simulink model "Simulink_6"  (R2016b)
settings: Solver=VariableStepAuto  StartTime=0.0  StopTime=70  RelTol=1e-3
values from neighbouring files (symbols this model uses):
  C_lon = [1 0 0 0 ... (first row only)    [ejercicio07_longitudinal_C.m]
  D_lon = zeros(2)    [ejercicio07_longitudinal_C.m]
  delta_e_dot_lim = [-90 90]    [ejercicio07_lateral_C.m]    (also in ejercicio07_longitudinal_C.m)
  delta_e_lim = [-25 25]    [ejercicio07_lateral_C.m]    (also in ejercicio07_longitudinal_C.m)
  delta_th_dot_lim = [-0.24 0.24]*100    [ejercicio07_lateral_C.m]    (also in ejercicio07_longitudinal_C.m)
  delta_th_lim = [-0.2 0.8]*100    [ejercicio07_lateral_C.m]    (also in ejercicio07_longitudinal_C.m)
  dt = 0.001    [ejercicio07_lateral_C.m]    (also in ejercicio07_longitudinal_C.m)
  F_lon = A_lon*Tm + I    [ejercicio07_longitudinal_C.m]
  G_lon = B_lon*Tm    [ejercicio07_longitudinal_C.m]
  Kc = Kc_a(:,1:4)    [ejercicio07_lateral_C.m]    (also in ejercicio07_longitudinal_C.m)
  Ki = -Kc_a(:,5:6)    [ejercicio07_lateral_C.m]    (also in ejercicio07_longitudinal_C.m)
  Ko_d = dlqe(F_lat,G_lat,C_lat,V1,V2)    [ejercicio07_lateral_C.m]    (also in ejercicio07_longitudinal_C.m = dlqe(F_lon,G_lon,C_lon,V1,V2))
  PreC = [Cyr*(I-Fyr)^(-1)*G_lat+D_lat]^(-1)    [ejercicio07_lateral_C.m]    (also in ejercicio07_longitudinal_C.m = [Cyr*(I-Fyr)^(-1)*G_lon+D_lon]^(-1))
  tau_e = 1/20    (= 0.05)    [ejercicio07_longitudinal_C.m]
  tau_th = 0.5    [ejercicio07_longitudinal_C.m]
  Tm = 0.003    [ejercicio07_lateral_C.m]    (also in ejercicio07_longitudinal_C.m)
undefined symbols (not defined in the file or in its folder): DiscIntNeverNeededParam, Ko
undefined symbols (not defined in the file): sys_lon
(part 2 of 3)

== system Simulink_6/Ejercicio 6/EJERCICIO 6 DISCRETO/Comparativa ejercicio 6/Comparativa Integral/CONTROL LONGITUDINAL CONTINUO ACCION INTEGRAL ==
  ACTUADORES : Subsystem
  Add : Sum  Inputs=+
  Add1 : Sum  Inputs=+
  Add2 : Sum  Inputs=+
  DINAMICA LONGITUDINAL : Subsystem  mask(Dinámica longitudinal F-16){A=sys_lon.a, B=sys_lon.b, C=sys_lon.c, D=sys_lon.d, X0=[0 0 0 0]}
      mask prompts: A "Matriz de estados (A)"; B "Matriz de entrada (B)"; C "Matriz de salida (C)"; D "Matriz de transmisión directa (D)"; X0 "Condiciones iniciales (nominales)"
      mask help: Modelo lineal de la dinámica longitudinal del F-16
  FILTRO SP : Subsystem
  Gain1 : Gain  Gain=PreC  Multiplication=Matrix(K*u)
  KT/taup2 : Gain  Gain=Kc  Multiplication=Matrix(K*u)
  Mux : Mux  Inputs=2
  OBSERVADOR : Subsystem  mask(Dinámica longitudinal F-16){A=sys_lon.a, B=sys_lon.b, C=sys_lon.c, D=sys_lon.d, X0=[0 0 0 0], Ko=Ko}
      mask prompts: A "Matriz de estados (A)"; B "Matriz de entrada (B)"; C "Matriz de salida (C)"; D "Matriz de transmisión directa (D)"; X0 "Condiciones iniciales (nominales)"; Ko "Ganancia del observador"
      mask help: Modelo lineal de la dinámica longitudinal del F-16
  Perturbación1 : Step  Time=[45 46]  After=[1 -1]*3  SampleTime=0
  SENSORES : Subsystem
  Sum1 : Sum  Inputs=|+-
  Sum2 : Sum  Inputs=|++
  Sum3 : Sum  Inputs=|+-
  Transfer Fcn : TransferFcn  Denominator=[1 1]
  thetaSP1 : Step  Time=[35,40]  Before=[0,0]  After=[5,5]  SampleTime=0
  vT_SP1 : Step  Time=[1,20]  Before=[0,0]  After=[30,15]  SampleTime=0
  CONTINUA : Outport
  wires:
  Add1/1 -> FILTRO SP/1(vt-sp)
  Gain1/1 -> Sum1/1
  Add2/1 -> FILTRO SP/2(theta_sp)
  thetaSP1/1 -> Add2/1
  DINAMICA LONGITUDINAL/1(y) -> Mux/1, SENSORES/1(y)  "y"
  [SP] -> Mux/2
  SENSORES/1(ym) -> OBSERVADOR/2(y), Sum3/2
  Mux/1 -> CONTINUA/1
  Perturbación1/1 -> Add/1
  OBSERVADOR/1(xest) -> KT/taup2/1
  Sum1/1 -> ACTUADORES/1(e)
  vT_SP1/1 -> Add1/1
  ACTUADORES/1(u) -> OBSERVADOR/1(u), Sum2/2
  Sum2/1 -> DINAMICA LONGITUDINAL/1(u)
  KT/taup2/1 -> Sum1/2
  Add/1 -> Transfer Fcn/1
  Transfer Fcn/1 -> Sum2/1
  Sum3/1 -> Gain1/1
  FILTRO SP/1(sp) -> Sum3/1, [SP]

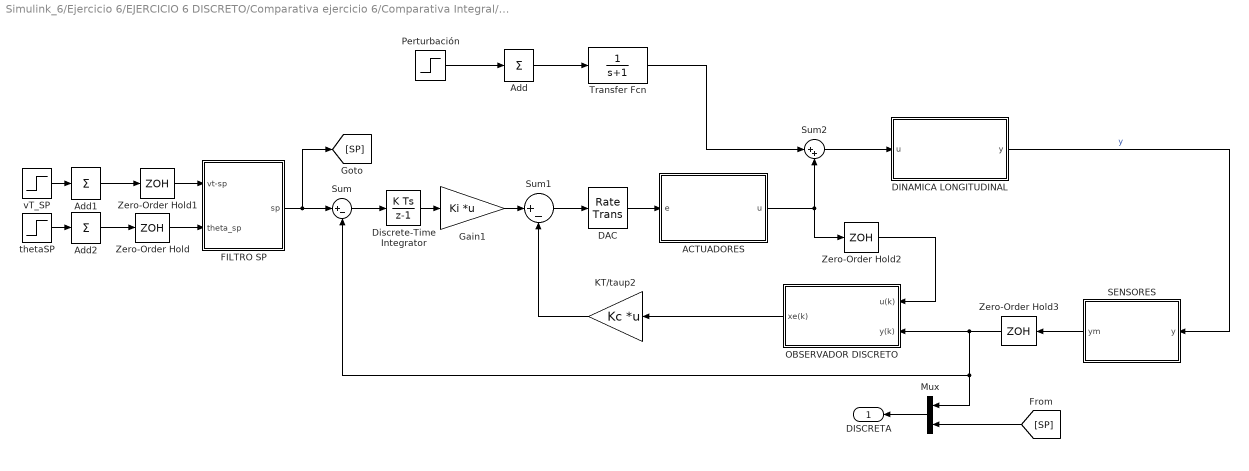
== system Simulink_6/Ejercicio 6/EJERCICIO 6 DISCRETO/Comparativa ejercicio 6/Comparativa Integral/CONTROL LONGITUDINAL DISCRETO ACCION INTEGRAL ==
  ACTUADORES : Subsystem
  Add : Sum  Inputs=+
  Add1 : Sum  Inputs=+
  Add2 : Sum  Inputs=+
  DAC : RateTransition  OutPortSampleTime=Tm
  DINAMICA LONGITUDINAL : Subsystem  mask(Dinámica longitudinal F-16){A=sys_lon.a, B=sys_lon.b, C=sys_lon.c, D=sys_lon.d, X0=[0 0 0 0]}
      mask prompts: A "Matriz de estados (A)"; B "Matriz de entrada (B)"; C "Matriz de salida (C)"; D "Matriz de transmisión directa (D)"; X0 "Condiciones iniciales (nominales)"
      mask help: Modelo lineal de la dinámica longitudinal del F-16
  Discrete-Time Integrator : DiscreteIntegrator  InitialConditionSetting=State (most efficient)  SampleTime=-1  ICPrevOutput=DiscIntNeverNeededParam  ICPrevScaledInput=DiscIntNeverNeededParam
  FILTRO SP : Subsystem
  Gain1 : Gain  Gain=Ki  Multiplication=Matrix(K*u)
  KT/taup2 : Gain  Gain=Kc  Multiplication=Matrix(K*u)
  Mux : Mux  Inputs=2
  OBSERVADOR DISCRETO : Subsystem  mask(Dinámica longitudinal F-16){F=F_lon, G=G_lon, C=C_lon, D=D_lon, Ko=Ko_d}
      mask prompts: F "Matriz de estados (A)"; G "Matriz de entrada (B)"; C "Matriz de salida (C)"; D "Matriz de transmisión directa (D)"; Ko "Ganancia del observador"
      mask help: Modelo lineal de la dinámica longitudinal del F-16
  Perturbación : Step  Time=[45 46]  After=[1 -1]*3  SampleTime=0
  SENSORES : Subsystem
  Sum : Sum  Inputs=|+-
  Sum1 : Sum  Inputs=|+-
  Sum2 : Sum  Inputs=|++
  Transfer Fcn : TransferFcn  Denominator=[1 1]
  Zero-Order Hold{,1..3} (4 alike) : ZeroOrderHold  SampleTime=-1
  thetaSP : Step  Time=[35,40]  Before=[0,0]  After=[5,5]  SampleTime=0
  vT_SP : Step  Time=[1,20]  Before=[0,0]  After=[30,15]  SampleTime=0
  DISCRETA : Outport
  wires:
  Zero-Order Hold/1 -> FILTRO SP/2(theta_sp)
  ACTUADORES/1(u) -> Sum2/2, Zero-Order Hold2/1
  Add/1 -> Transfer Fcn/1
  FILTRO SP/1(sp) -> Sum/1, [SP]
  DAC/1 -> ACTUADORES/1(e)
  Mux/1 -> DISCRETA/1
  OBSERVADOR DISCRETO/1(xe(k)) -> KT/taup2/1
  DINAMICA LONGITUDINAL/1(y) -> SENSORES/1(y)  "y"
  Transfer Fcn/1 -> Sum2/1
  KT/taup2/1 -> Sum1/2
  Zero-Order Hold2/1 -> OBSERVADOR DISCRETO/1(u(k))
  SENSORES/1(ym) -> Zero-Order Hold3/1
  Zero-Order Hold3/1 -> OBSERVADOR DISCRETO/2(y(k)), Sum/2, Mux/1
  [SP] -> Mux/2
  Add1/1 -> Zero-Order Hold1/1
  Add2/1 -> Zero-Order Hold/1
  Sum2/1 -> DINAMICA LONGITUDINAL/1(u)
  Sum1/1 -> DAC/1
  Zero-Order Hold1/1 -> FILTRO SP/1(vt-sp)
  vT_SP/1 -> Add1/1
  Perturbación/1 -> Add/1
  thetaSP/1 -> Add2/1
  Gain1/1 -> Sum1/1
  Sum/1 -> Discrete-Time Integrator/1
  Discrete-Time Integrator/1 -> Gain1/1

== system Simulink_6/Ejercicio 6/EJERCICIO 6 DISCRETO/Comparativa ejercicio 6/Comparativa modal/CONTROL LONGITUDINAL CONTINUA ==
  ACTUADORES : Subsystem
  Add : Sum  Inputs=+
  Add1 : Sum  Inputs=+
  Add2 : Sum  Inputs=+
  DINAMICA LONGITUDINAL : Subsystem  mask(Dinámica longitudinal F-16){A=sys_lon.a, B=sys_lon.b, C=sys_lon.c, D=sys_lon.d, X0=[0 0 0 0]}
      mask prompts: A "Matriz de estados (A)"; B "Matriz de entrada (B)"; C "Matriz de salida (C)"; D "Matriz de transmisión directa (D)"; X0 "Condiciones iniciales (nominales)"
      mask help: Modelo lineal de la dinámica longitudinal del F-16
  FILTRO SP : Subsystem
  Gain1 : Gain  Gain=PreC  Multiplication=Matrix(K*u)
  KT/taup2 : Gain  Gain=Kc  Multiplication=Matrix(K*u)
  Mux : Mux  Inputs=2
  OBSERVADOR : Subsystem  mask(Dinámica longitudinal F-16){A=sys_lon.a, B=sys_lon.b, C=sys_lon.c, D=sys_lon.d, X0=[0 0 0 0], Ko=Ko}
      mask prompts: A "Matriz de estados (A)"; B "Matriz de entrada (B)"; C "Matriz de salida (C)"; D "Matriz de transmisión directa (D)"; X0 "Condiciones iniciales (nominales)"; Ko "Ganancia del observador"
      mask help: Modelo lineal de la dinámica longitudinal del F-16
  Perturbación1 : Step  Time=[45 46]  After=[1 -1]*3  SampleTime=0
  SENSORES : Subsystem
  Sum1 : Sum  Inputs=|+-
  Sum2 : Sum  Inputs=|++
  Transfer Fcn : TransferFcn  Denominator=[1 1]
  thetaSP1 : Step  Time=[35,40]  Before=[0,0]  After=[5,5]  SampleTime=0
  vT_SP1 : Step  Time=[1,20]  Before=[0,0]  After=[30,15]  SampleTime=0
  CONTINUA : Outport
  wires:
  OBSERVADOR/1(xest) -> KT/taup2/1
  [SP] -> Mux/2
  vT_SP1/1 -> Add1/1
  Add2/1 -> FILTRO SP/2(theta_sp)
  thetaSP1/1 -> Add2/1
  Sum1/1 -> ACTUADORES/1(e)
  DINAMICA LONGITUDINAL/1(y) -> Mux/1, SENSORES/1(y)  "y"
  SENSORES/1(ym) -> OBSERVADOR/2(y)
  Gain1/1 -> Sum1/1
  KT/taup2/1 -> Sum1/2
  Add1/1 -> FILTRO SP/1(vt-sp)
  Add/1 -> Transfer Fcn/1
  Perturbación1/1 -> Add/1
  Sum2/1 -> DINAMICA LONGITUDINAL/1(u)
  Transfer Fcn/1 -> Sum2/1
  ACTUADORES/1(u) -> OBSERVADOR/1(u), Sum2/2
  FILTRO SP/1(sp) -> Gain1/1, [SP]
  Mux/1 -> CONTINUA/1

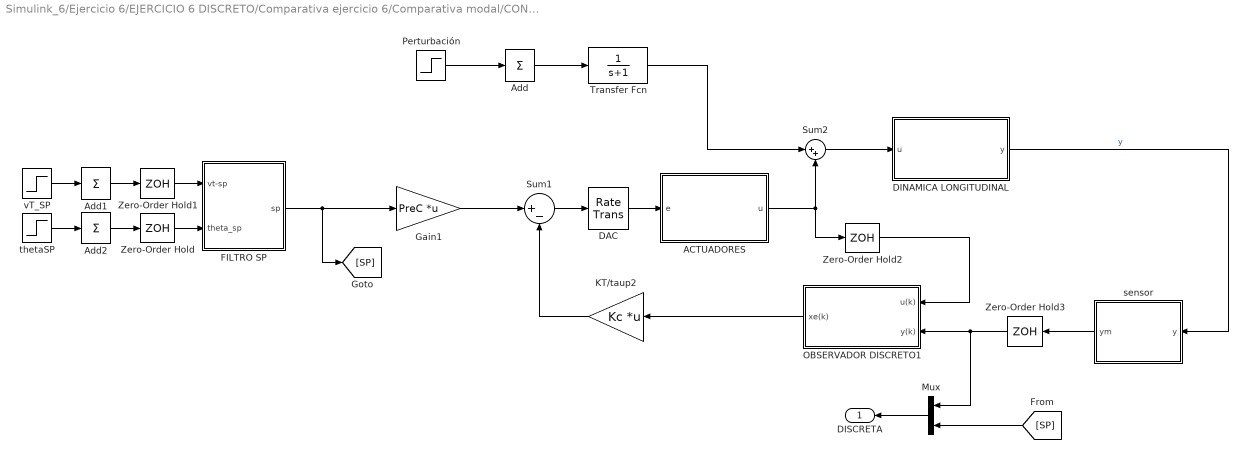
== system Simulink_6/Ejercicio 6/EJERCICIO 6 DISCRETO/Comparativa ejercicio 6/Comparativa modal/CONTROL LONGITUDINAL DISCRETO ==
  ACTUADORES : Subsystem
  Add : Sum  Inputs=+
  Add1 : Sum  Inputs=+
  Add2 : Sum  Inputs=+
  DAC : RateTransition  OutPortSampleTime=Tm
  DINAMICA LONGITUDINAL : Subsystem  mask(Dinámica longitudinal F-16){A=sys_lon.a, B=sys_lon.b, C=sys_lon.c, D=sys_lon.d, X0=[0 0 0 0]}
      mask prompts: A "Matriz de estados (A)"; B "Matriz de entrada (B)"; C "Matriz de salida (C)"; D "Matriz de transmisión directa (D)"; X0 "Condiciones iniciales (nominales)"
      mask help: Modelo lineal de la dinámica longitudinal del F-16
  FILTRO SP : Subsystem
  Gain1 : Gain  Gain=PreC  Multiplication=Matrix(K*u)
  KT/taup2 : Gain  Gain=Kc  Multiplication=Matrix(K*u)
  Mux : Mux  Inputs=2
  OBSERVADOR DISCRETO1 : Subsystem  mask(Dinámica longitudinal F-16){F=F_lon, G=G_lon, C=C_lon, D=D_lon, Ko=Ko_d}
      mask prompts: F "Matriz de estados (A)"; G "Matriz de entrada (B)"; C "Matriz de salida (C)"; D "Matriz de transmisión directa (D)"; Ko "Ganancia del observador"
      mask help: Modelo lineal de la dinámica longitudinal del F-16
  Perturbación : Step  Time=[45 46]  After=[1 -1]*3  SampleTime=0
  Sum1 : Sum  Inputs=|+-
  Sum2 : Sum  Inputs=|++
  Transfer Fcn : TransferFcn  Denominator=[1 1]
  Zero-Order Hold{,1..3} (4 alike) : ZeroOrderHold  SampleTime=-1
  sensor : Subsystem
  thetaSP : Step  Time=[35,40]  Before=[0,0]  After=[5,5]  SampleTime=0
  vT_SP : Step  Time=[1,20]  Before=[0,0]  After=[30,15]  SampleTime=0
  DISCRETA : Outport
  wires:
  KT/taup2/1 -> Sum1/2
  FILTRO SP/1(sp) -> Gain1/1, [SP]
  Gain1/1 -> Sum1/1
  OBSERVADOR DISCRETO1/1(xe(k)) -> KT/taup2/1
  Mux/1 -> DISCRETA/1
  [SP] -> Mux/2
  ACTUADORES/1(u) -> Zero-Order Hold2/1, Sum2/2
  Sum2/1 -> DINAMICA LONGITUDINAL/1(u)
  Transfer Fcn/1 -> Sum2/1
  Add/1 -> Transfer Fcn/1
  Perturbación/1 -> Add/1
  thetaSP/1 -> Add2/1
  vT_SP/1 -> Add1/1
  Add2/1 -> Zero-Order Hold/1
  Zero-Order Hold1/1 -> FILTRO SP/1(vt-sp)
  Add1/1 -> Zero-Order Hold1/1
  Zero-Order Hold/1 -> FILTRO SP/2(theta_sp)
  DAC/1 -> ACTUADORES/1(e)
  Sum1/1 -> DAC/1
  Zero-Order Hold2/1 -> OBSERVADOR DISCRETO1/1(u(k))
  DINAMICA LONGITUDINAL/1(y) -> sensor/1(y)  "y"
  sensor/1(ym) -> Zero-Order Hold3/1
  Zero-Order Hold3/1 -> OBSERVADOR DISCRETO1/2(y(k)), Mux/1

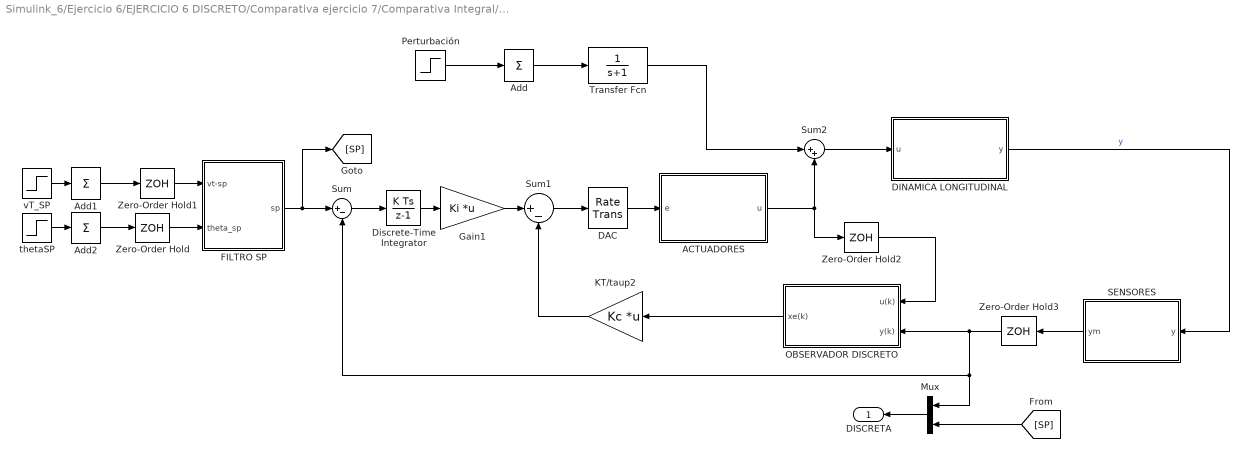
== system Simulink_6/Ejercicio 6/EJERCICIO 6 DISCRETO/Comparativa ejercicio 7/Comparativa Integral/CONTROL LONGITUDINAL DISCRETO ACCION INTEGRAL ==
  ACTUADORES : Subsystem
  Add : Sum  Inputs=+
  Add1 : Sum  Inputs=+
  Add2 : Sum  Inputs=+
  DAC : RateTransition  OutPortSampleTime=Tm
  DINAMICA LONGITUDINAL : Subsystem  mask(Dinámica longitudinal F-16){A=sys_lon.a, B=sys_lon.b, C=sys_lon.c, D=sys_lon.d, X0=[0 0 0 0]}
      mask prompts: A "Matriz de estados (A)"; B "Matriz de entrada (B)"; C "Matriz de salida (C)"; D "Matriz de transmisión directa (D)"; X0 "Condiciones iniciales (nominales)"
      mask help: Modelo lineal de la dinámica longitudinal del F-16
  Discrete-Time Integrator : DiscreteIntegrator  InitialConditionSetting=State (most efficient)  SampleTime=-1  ICPrevOutput=DiscIntNeverNeededParam  ICPrevScaledInput=DiscIntNeverNeededParam
  FILTRO SP : Subsystem
  Gain1 : Gain  Gain=Ki  Multiplication=Matrix(K*u)
  KT/taup2 : Gain  Gain=Kc  Multiplication=Matrix(K*u)
  Mux : Mux  Inputs=2
  OBSERVADOR DISCRETO : Subsystem  mask(Dinámica longitudinal F-16){F=F_lon, G=G_lon, C=C_lon, D=D_lon, Ko=Ko_d}
      mask prompts: F "Matriz de estados (A)"; G "Matriz de entrada (B)"; C "Matriz de salida (C)"; D "Matriz de transmisión directa (D)"; Ko "Ganancia del observador"
      mask help: Modelo lineal de la dinámica longitudinal del F-16
  Perturbación : Step  Time=[45 46]  After=[1 -1]*3  SampleTime=0
  SENSORES : Subsystem
  Sum : Sum  Inputs=|+-
  Sum1 : Sum  Inputs=|+-
  Sum2 : Sum  Inputs=|++
  Transfer Fcn : TransferFcn  Denominator=[1 1]
  Zero-Order Hold{,1..3} (4 alike) : ZeroOrderHold  SampleTime=-1
  thetaSP : Step  Time=[35,40]  Before=[0,0]  After=[5,5]  SampleTime=0
  vT_SP : Step  Time=[1,20]  Before=[0,0]  After=[30,15]  SampleTime=0
  DISCRETA : Outport
  wires:
  Zero-Order Hold/1 -> FILTRO SP/2(theta_sp)
  ACTUADORES/1(u) -> Sum2/2, Zero-Order Hold2/1
  Add/1 -> Transfer Fcn/1
  FILTRO SP/1(sp) -> Sum/1, [SP]
  DAC/1 -> ACTUADORES/1(e)
  Mux/1 -> DISCRETA/1
  OBSERVADOR DISCRETO/1(xe(k)) -> KT/taup2/1
  DINAMICA LONGITUDINAL/1(y) -> SENSORES/1(y)  "y"
  Transfer Fcn/1 -> Sum2/1
  KT/taup2/1 -> Sum1/2
  Zero-Order Hold2/1 -> OBSERVADOR DISCRETO/1(u(k))
  SENSORES/1(ym) -> Zero-Order Hold3/1
  Zero-Order Hold3/1 -> OBSERVADOR DISCRETO/2(y(k)), Sum/2, Mux/1
  [SP] -> Mux/2
  Add1/1 -> Zero-Order Hold1/1
  Add2/1 -> Zero-Order Hold/1
  Sum2/1 -> DINAMICA LONGITUDINAL/1(u)
  Sum1/1 -> DAC/1
  Zero-Order Hold1/1 -> FILTRO SP/1(vt-sp)
  vT_SP/1 -> Add1/1
  Perturbación/1 -> Add/1
  thetaSP/1 -> Add2/1
  Gain1/1 -> Sum1/1
  Sum/1 -> Discrete-Time Integrator/1
  Discrete-Time Integrator/1 -> Gain1/1

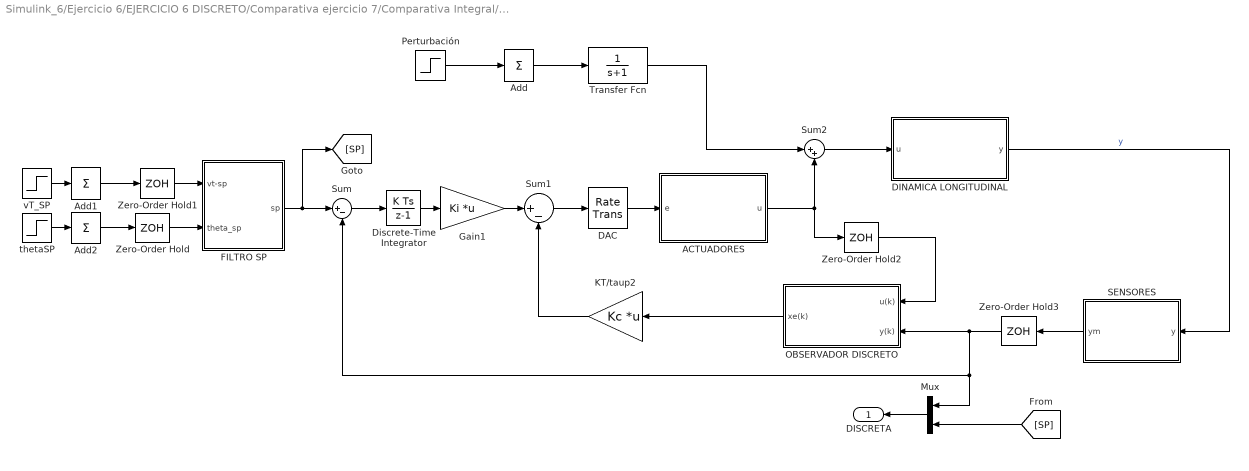
== system Simulink_6/Ejercicio 6/EJERCICIO 6 DISCRETO/Comparativa ejercicio 7/Comparativa Integral/CONTROL LONGITUDINAL DISCRETO ACCION INTEGRAL1 ==
  ACTUADORES : Subsystem
  Add : Sum  Inputs=+
  Add1 : Sum  Inputs=+
  Add2 : Sum  Inputs=+
  DAC : RateTransition  OutPortSampleTime=Tm
  DINAMICA LONGITUDINAL : Subsystem  mask(Dinámica longitudinal F-16){A=sys_lon.a, B=sys_lon.b, C=sys_lon.c, D=sys_lon.d, X0=[0 0 0 0]}
      mask prompts: A "Matriz de estados (A)"; B "Matriz de entrada (B)"; C "Matriz de salida (C)"; D "Matriz de transmisión directa (D)"; X0 "Condiciones iniciales (nominales)"
      mask help: Modelo lineal de la dinámica longitudinal del F-16
  Discrete-Time Integrator : DiscreteIntegrator  InitialConditionSetting=State (most efficient)  SampleTime=-1  ICPrevOutput=DiscIntNeverNeededParam  ICPrevScaledInput=DiscIntNeverNeededParam
  FILTRO SP : Subsystem
  Gain1 : Gain  Gain=Ki  Multiplication=Matrix(K*u)
  KT/taup2 : Gain  Gain=Kc  Multiplication=Matrix(K*u)
  Mux : Mux  Inputs=2
  OBSERVADOR DISCRETO : Subsystem  mask(Dinámica longitudinal F-16){F=F_lon, G=G_lon, C=C_lon, D=D_lon, Ko=Ko_d}
      mask prompts: F "Matriz de estados (A)"; G "Matriz de entrada (B)"; C "Matriz de salida (C)"; D "Matriz de transmisión directa (D)"; Ko "Ganancia del observador"
      mask help: Modelo lineal de la dinámica longitudinal del F-16
  Perturbación : Step  Time=[45 46]  After=[1 -1]*3  SampleTime=0
  SENSORES : Subsystem
  Sum : Sum  Inputs=|+-
  Sum1 : Sum  Inputs=|+-
  Sum2 : Sum  Inputs=|++
  Transfer Fcn : TransferFcn  Denominator=[1 1]
  Zero-Order Hold{,1..3} (4 alike) : ZeroOrderHold  SampleTime=-1
  thetaSP : Step  Time=[35,40]  Before=[0,0]  After=[5,5]  SampleTime=0
  vT_SP : Step  Time=[1,20]  Before=[0,0]  After=[30,15]  SampleTime=0
  DISCRETA : Outport
  wires:
  Zero-Order Hold/1 -> FILTRO SP/2(theta_sp)
  ACTUADORES/1(u) -> Sum2/2, Zero-Order Hold2/1
  Add/1 -> Transfer Fcn/1
  FILTRO SP/1(sp) -> Sum/1, [SP]
  DAC/1 -> ACTUADORES/1(e)
  Mux/1 -> DISCRETA/1
  OBSERVADOR DISCRETO/1(xe(k)) -> KT/taup2/1
  DINAMICA LONGITUDINAL/1(y) -> SENSORES/1(y)  "y"
  Transfer Fcn/1 -> Sum2/1
  KT/taup2/1 -> Sum1/2
  Zero-Order Hold2/1 -> OBSERVADOR DISCRETO/1(u(k))
  SENSORES/1(ym) -> Zero-Order Hold3/1
  Zero-Order Hold3/1 -> OBSERVADOR DISCRETO/2(y(k)), Sum/2, Mux/1
  [SP] -> Mux/2
  Add1/1 -> Zero-Order Hold1/1
  Add2/1 -> Zero-Order Hold/1
  Sum2/1 -> DINAMICA LONGITUDINAL/1(u)
  Sum1/1 -> DAC/1
  Zero-Order Hold1/1 -> FILTRO SP/1(vt-sp)
  vT_SP/1 -> Add1/1
  Perturbación/1 -> Add/1
  thetaSP/1 -> Add2/1
  Gain1/1 -> Sum1/1
  Sum/1 -> Discrete-Time Integrator/1
  Discrete-Time Integrator/1 -> Gain1/1

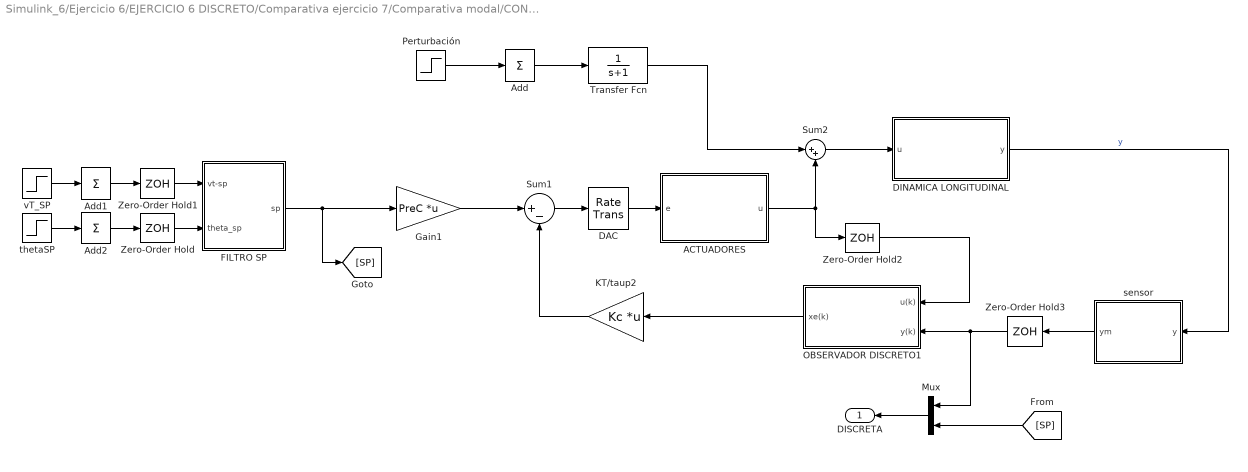
== system Simulink_6/Ejercicio 6/EJERCICIO 6 DISCRETO/Comparativa ejercicio 7/Comparativa modal/CONTROL LONGITUDINAL DISCRETO EJERCICIO 6 ==
  ACTUADORES : Subsystem
  Add : Sum  Inputs=+
  Add1 : Sum  Inputs=+
  Add2 : Sum  Inputs=+
  DAC : RateTransition  OutPortSampleTime=Tm
  DINAMICA LONGITUDINAL : Subsystem  mask(Dinámica longitudinal F-16){A=sys_lon.a, B=sys_lon.b, C=sys_lon.c, D=sys_lon.d, X0=[0 0 0 0]}
      mask prompts: A "Matriz de estados (A)"; B "Matriz de entrada (B)"; C "Matriz de salida (C)"; D "Matriz de transmisión directa (D)"; X0 "Condiciones iniciales (nominales)"
      mask help: Modelo lineal de la dinámica longitudinal del F-16
  FILTRO SP : Subsystem
  Gain1 : Gain  Gain=PreC  Multiplication=Matrix(K*u)
  KT/taup2 : Gain  Gain=Kc  Multiplication=Matrix(K*u)
  Mux : Mux  Inputs=2
  OBSERVADOR DISCRETO1 : Subsystem  mask(Dinámica longitudinal F-16){F=F_lon, G=G_lon, C=C_lon, D=D_lon, Ko=Ko_d}
      mask prompts: F "Matriz de estados (A)"; G "Matriz de entrada (B)"; C "Matriz de salida (C)"; D "Matriz de transmisión directa (D)"; Ko "Ganancia del observador"
      mask help: Modelo lineal de la dinámica longitudinal del F-16
  Perturbación : Step  Time=[45 46]  After=[1 -1]*3  SampleTime=0
  Sum1 : Sum  Inputs=|+-
  Sum2 : Sum  Inputs=|++
  Transfer Fcn : TransferFcn  Denominator=[1 1]
  Zero-Order Hold{,1..3} (4 alike) : ZeroOrderHold  SampleTime=-1
  sensor : Subsystem
  thetaSP : Step  Time=[35,40]  Before=[0,0]  After=[5,5]  SampleTime=0
  vT_SP : Step  Time=[1,20]  Before=[0,0]  After=[30,15]  SampleTime=0
  DISCRETA : Outport
  wires:
  KT/taup2/1 -> Sum1/2
  FILTRO SP/1(sp) -> Gain1/1, [SP]
  Gain1/1 -> Sum1/1
  OBSERVADOR DISCRETO1/1(xe(k)) -> KT/taup2/1
  Mux/1 -> DISCRETA/1
  [SP] -> Mux/2
  ACTUADORES/1(u) -> Zero-Order Hold2/1, Sum2/2
  Sum2/1 -> DINAMICA LONGITUDINAL/1(u)
  Transfer Fcn/1 -> Sum2/1
  Add/1 -> Transfer Fcn/1
  Perturbación/1 -> Add/1
  thetaSP/1 -> Add2/1
  vT_SP/1 -> Add1/1
  Add2/1 -> Zero-Order Hold/1
  Zero-Order Hold1/1 -> FILTRO SP/1(vt-sp)
  Add1/1 -> Zero-Order Hold1/1
  Zero-Order Hold/1 -> FILTRO SP/2(theta_sp)
  DAC/1 -> ACTUADORES/1(e)
  Sum1/1 -> DAC/1
  Zero-Order Hold2/1 -> OBSERVADOR DISCRETO1/1(u(k))
  DINAMICA LONGITUDINAL/1(y) -> sensor/1(y)  "y"
  sensor/1(ym) -> Zero-Order Hold3/1
  Zero-Order Hold3/1 -> OBSERVADOR DISCRETO1/2(y(k)), Mux/1

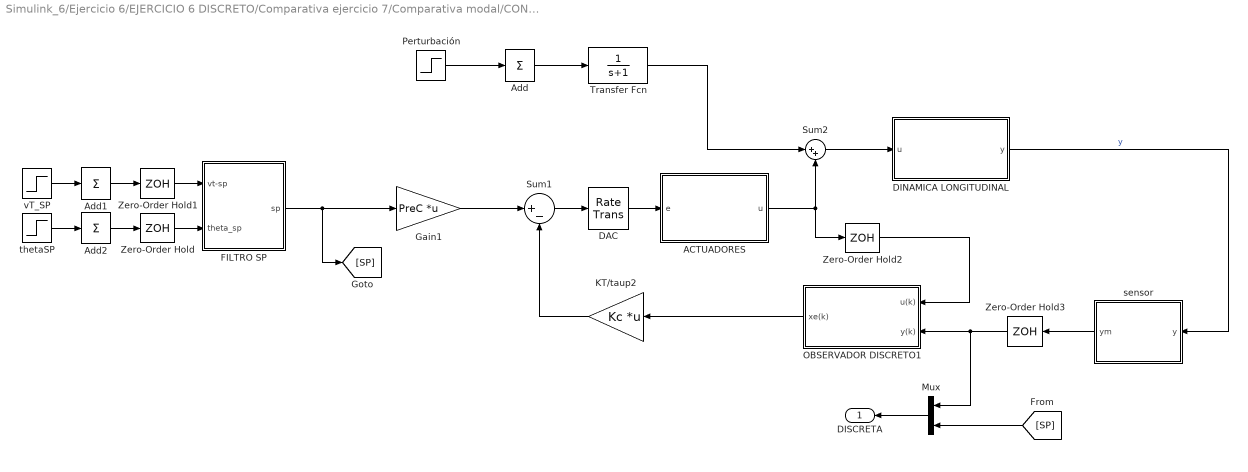
== system Simulink_6/Ejercicio 6/EJERCICIO 6 DISCRETO/Comparativa ejercicio 7/Comparativa modal/CONTROL LONGITUDINAL DISCRETO EJERCICIO 7 ==
  ACTUADORES : Subsystem
  Add : Sum  Inputs=+
  Add1 : Sum  Inputs=+
  Add2 : Sum  Inputs=+
  DAC : RateTransition  OutPortSampleTime=Tm
  DINAMICA LONGITUDINAL : Subsystem  mask(Dinámica longitudinal F-16){A=sys_lon.a, B=sys_lon.b, C=sys_lon.c, D=sys_lon.d, X0=[0 0 0 0]}
      mask prompts: A "Matriz de estados (A)"; B "Matriz de entrada (B)"; C "Matriz de salida (C)"; D "Matriz de transmisión directa (D)"; X0 "Condiciones iniciales (nominales)"
      mask help: Modelo lineal de la dinámica longitudinal del F-16
  FILTRO SP : Subsystem
  Gain1 : Gain  Gain=PreC  Multiplication=Matrix(K*u)
  KT/taup2 : Gain  Gain=Kc  Multiplication=Matrix(K*u)
  Mux : Mux  Inputs=2
  OBSERVADOR DISCRETO1 : Subsystem  mask(Dinámica longitudinal F-16){F=F_lon, G=G_lon, C=C_lon, D=D_lon, Ko=Ko_d}
      mask prompts: F "Matriz de estados (A)"; G "Matriz de entrada (B)"; C "Matriz de salida (C)"; D "Matriz de transmisión directa (D)"; Ko "Ganancia del observador"
      mask help: Modelo lineal de la dinámica longitudinal del F-16
  Perturbación : Step  Time=[45 46]  After=[1 -1]*3  SampleTime=0
  Sum1 : Sum  Inputs=|+-
  Sum2 : Sum  Inputs=|++
  Transfer Fcn : TransferFcn  Denominator=[1 1]
  Zero-Order Hold{,1..3} (4 alike) : ZeroOrderHold  SampleTime=-1
  sensor : Subsystem
  thetaSP : Step  Time=[35,40]  Before=[0,0]  After=[5,5]  SampleTime=0
  vT_SP : Step  Time=[1,20]  Before=[0,0]  After=[30,15]  SampleTime=0
  DISCRETA : Outport
  wires:
  KT/taup2/1 -> Sum1/2
  FILTRO SP/1(sp) -> Gain1/1, [SP]
  Gain1/1 -> Sum1/1
  OBSERVADOR DISCRETO1/1(xe(k)) -> KT/taup2/1
  Mux/1 -> DISCRETA/1
  [SP] -> Mux/2
  ACTUADORES/1(u) -> Zero-Order Hold2/1, Sum2/2
  Sum2/1 -> DINAMICA LONGITUDINAL/1(u)
  Transfer Fcn/1 -> Sum2/1
  Add/1 -> Transfer Fcn/1
  Perturbación/1 -> Add/1
  thetaSP/1 -> Add2/1
  vT_SP/1 -> Add1/1
  Add2/1 -> Zero-Order Hold/1
  Zero-Order Hold1/1 -> FILTRO SP/1(vt-sp)
  Add1/1 -> Zero-Order Hold1/1
  Zero-Order Hold/1 -> FILTRO SP/2(theta_sp)
  DAC/1 -> ACTUADORES/1(e)
  Sum1/1 -> DAC/1
  Zero-Order Hold2/1 -> OBSERVADOR DISCRETO1/1(u(k))
  DINAMICA LONGITUDINAL/1(y) -> sensor/1(y)  "y"
  sensor/1(ym) -> Zero-Order Hold3/1
  Zero-Order Hold3/1 -> OBSERVADOR DISCRETO1/2(y(k)), Mux/1

== system Simulink_6/Ejercicio 6/EJERCICIO 6 DISCRETO/Comparativa ejercicio 6/Comparativa Integral/CONTROL LONGITUDINAL CONTINUO ACCION INTEGRAL/ACTUADORES ==
  e : Inport
  Actuadores : Scope
  Demux : Demux  Outputs=2
  ELEVADOR : Subsystem
  Gain4 : Gain  Gain=[1 180/pi]
  Mux1 : Mux  Inputs=2
  THROTTLE : Subsystem
  u : Outport
  wires:
  Demux/1 -> THROTTLE/1(u_th)
  Demux/2 -> ELEVADOR/1(u_e)
  ELEVADOR/1(delta_e) -> Mux1/2
  e/1 -> Demux/1
  Mux1/1 -> u/1, Gain4/1
  Gain4/1 -> Actuadores/1
  THROTTLE/1(delta_th) -> Mux1/1

== system Simulink_6/Ejercicio 6/EJERCICIO 6 DISCRETO/Comparativa ejercicio 6/Comparativa Integral/CONTROL LONGITUDINAL CONTINUO ACCION INTEGRAL/DINAMICA LONGITUDINAL ==
  u : Inport
  Integrator5 : Integrator
  Km1 : Gain  Gain=D  Multiplication=Matrix(K*u)
  Km10 : Gain  Gain=A  Multiplication=Matrix(K*u)
  Km2 : Gain  Gain=C  Multiplication=Matrix(K*u)
  Km8 : Gain  Gain=B  Multiplication=Matrix(K*u)
  Sum1 : Sum  Inputs=++|
  Sum12 : Sum  Inputs=|++
  y : Outport
  wires:
  Km8/1 -> Sum12/1
  Sum12/1 -> Integrator5/1
  Integrator5/1 -> Km2/1, Km10/1  "x"
  Km10/1 -> Sum12/2
  Km2/1 -> Sum1/2
  Km1/1 -> Sum1/1
  Sum1/1 -> y/1
  u/1 -> Km8/1, Km1/1

== system Simulink_6/Ejercicio 6/EJERCICIO 6 DISCRETO/Comparativa ejercicio 6/Comparativa Integral/CONTROL LONGITUDINAL CONTINUO ACCION INTEGRAL/FILTRO SP ==
  vt-sp : Inport
  theta_sp : Inport  Port=2
  Mux4 : Mux  Inputs=2
  Rate Limiter : RateLimiter  RisingSlewLimit=3  FallingSlewLimit=-3  SampleTimeMode=inherited
  Transfer Fcn : TransferFcn  Denominator=[1 1]
  sp : Outport
  wires:
  Rate Limiter/1 -> Transfer Fcn/1
  Transfer Fcn/1 -> Mux4/1
  vt-sp/1 -> Rate Limiter/1
  Mux4/1 -> sp/1
  theta_sp/1 -> Mux4/2

== system Simulink_6/Ejercicio 6/EJERCICIO 6 DISCRETO/Comparativa ejercicio 6/Comparativa Integral/CONTROL LONGITUDINAL CONTINUO ACCION INTEGRAL/OBSERVADOR ==
  u : Inport
  y : Inport  Port=2
  Integrator5 : Integrator
  Km1 : Gain  Gain=D  Multiplication=Matrix(K*u)
  Km10 : Gain  Gain=A  Multiplication=Matrix(K*u)
  Km2 : Gain  Gain=C  Multiplication=Matrix(K*u)
  Km3 : Gain  Gain=Ko  Multiplication=Matrix(K*u)
  Km8 : Gain  Gain=B  Multiplication=Matrix(K*u)
  Sum1 : Sum  Inputs=++|
  Sum12 : Sum  Inputs=+++
  Sum2 : Sum  Inputs=+-|
  xest : Outport
  wires:
  Km8/1 -> Sum12/1
  Sum12/1 -> Integrator5/1
  Integrator5/1 -> Km2/1, Km10/1, xest/1  "xe"
  Km10/1 -> Sum12/3
  Km2/1 -> Sum1/2
  Km1/1 -> Sum1/1
  Sum1/1 -> Sum2/2  "ye"
  u/1 -> Km8/1, Km1/1
  y/1 -> Sum2/1
  Sum2/1 -> Km3/1
  Km3/1 -> Sum12/2

== system Simulink_6/Ejercicio 6/EJERCICIO 6 DISCRETO/Comparativa ejercicio 6/Comparativa Integral/CONTROL LONGITUDINAL CONTINUO ACCION INTEGRAL/SENSORES ==
  y : Inport
  Add2 : Sum
  Add3 : Sum
  Demux : Demux  Outputs=2
  Mux2 : Mux  Inputs=2
  Ruido de medida1 : RandomNumber  Variance=1e-6  Seed=123456  SampleTime=dt
  Ruido de medida2 : RandomNumber  Variance=1e-6  Seed=123456  SampleTime=dt
  ym : Outport
  wires:
  y/1 -> Demux/1
  Ruido de medida1/1 -> Add2/1
  Add2/1 -> Mux2/1
  Demux/1 -> Add2/2
  Mux2/1 -> ym/1
  Demux/2 -> Add3/1
  Add3/1 -> Mux2/2
  Ruido de medida2/1 -> Add3/2

== system Simulink_6/Ejercicio 6/EJERCICIO 6 DISCRETO/Comparativa ejercicio 6/Comparativa Integral/CONTROL LONGITUDINAL DISCRETO ACCION INTEGRAL/ACTUADORES ==
  e : Inport
  Actuadores : Scope
  Demux : Demux  Outputs=2
  ELEVADOR : Subsystem
  Gain4 : Gain  Gain=[1 180/pi]
  Mux1 : Mux  Inputs=2
  THROTTLE : Subsystem
  u : Outport
  wires:
  Demux/1 -> THROTTLE/1(u_th)
  Demux/2 -> ELEVADOR/1(u_e)
  ELEVADOR/1(delta_e) -> Mux1/2
  e/1 -> Demux/1
  Mux1/1 -> u/1, Gain4/1
  Gain4/1 -> Actuadores/1
  THROTTLE/1(delta_th) -> Mux1/1

== system Simulink_6/Ejercicio 6/EJERCICIO 6 DISCRETO/Comparativa ejercicio 6/Comparativa Integral/CONTROL LONGITUDINAL DISCRETO ACCION INTEGRAL/DINAMICA LONGITUDINAL ==
  u : Inport
  Integrator5 : Integrator
  Km1 : Gain  Gain=D  Multiplication=Matrix(K*u)
  Km10 : Gain  Gain=A  Multiplication=Matrix(K*u)
  Km2 : Gain  Gain=C  Multiplication=Matrix(K*u)
  Km8 : Gain  Gain=B  Multiplication=Matrix(K*u)
  Sum1 : Sum  Inputs=++|
  Sum12 : Sum  Inputs=|++
  y : Outport
  wires:
  Km8/1 -> Sum12/1
  Sum12/1 -> Integrator5/1
  Integrator5/1 -> Km2/1, Km10/1  "x"
  Km10/1 -> Sum12/2
  Km2/1 -> Sum1/2
  Km1/1 -> Sum1/1
  Sum1/1 -> y/1
  u/1 -> Km8/1, Km1/1

== system Simulink_6/Ejercicio 6/EJERCICIO 6 DISCRETO/Comparativa ejercicio 6/Comparativa Integral/CONTROL LONGITUDINAL DISCRETO ACCION INTEGRAL/FILTRO SP ==
  vt-sp : Inport
  theta_sp : Inport  Port=2
  Discrete Transfer Fcn : DiscreteTransferFcn  Numerator=[Tm]  Denominator=[1 -1+Tm]
  Mux4 : Mux  Inputs=2
  Rate Limiter : RateLimiter  RisingSlewLimit=3  FallingSlewLimit=-3  SampleTimeMode=inherited
  sp : Outport
  wires:
  vt-sp/1 -> Rate Limiter/1
  Mux4/1 -> sp/1
  theta_sp/1 -> Mux4/2
  Rate Limiter/1 -> Discrete Transfer Fcn/1
  Discrete Transfer Fcn/1 -> Mux4/1

== system Simulink_6/Ejercicio 6/EJERCICIO 6 DISCRETO/Comparativa ejercicio 6/Comparativa Integral/CONTROL LONGITUDINAL DISCRETO ACCION INTEGRAL/OBSERVADOR DISCRETO ==
  u(k) : Inport
  y(k) : Inport  Port=2
  Km1 : Gain  Gain=D  Multiplication=Matrix(K*u)
  Km10 : Gain  Gain=F  Multiplication=Matrix(K*u)
  Km2 : Gain  Gain=C  Multiplication=Matrix(K*u)
  Km3 : Gain  Gain=Ko  Multiplication=Matrix(K*u)
  Km8 : Gain  Gain=G  Multiplication=Matrix(K*u)
  Sum1 : Sum  Inputs=++|
  Sum12 : Sum  Inputs=+++
  Sum2 : Sum  Inputs=+-|
  Unit Delay : UnitDelay  SampleTime=Tm  HasFrameUpgradeWarning=on
  xe(k) : Outport
  wires:
  Km8/1 -> Sum12/1
  Sum12/1 -> Unit Delay/1  "xe(k+1)"
  Unit Delay/1 -> Km2/1, Km10/1, xe(k)/1  "xe(k)"
  Km10/1 -> Sum12/3
  Km2/1 -> Sum1/2
  Km1/1 -> Sum1/1
  Sum1/1 -> Sum2/2  "ye(k)"
  u(k)/1 -> Km8/1, Km1/1
  y(k)/1 -> Sum2/1
  Sum2/1 -> Km3/1
  Km3/1 -> Sum12/2

== system Simulink_6/Ejercicio 6/EJERCICIO 6 DISCRETO/Comparativa ejercicio 6/Comparativa Integral/CONTROL LONGITUDINAL DISCRETO ACCION INTEGRAL/SENSORES ==
  y : Inport
  Add2 : Sum
  Add3 : Sum
  Demux : Demux  Outputs=2
  Mux2 : Mux  Inputs=2
  Ruido de medida1 : RandomNumber  Variance=1e-6  Seed=123456  SampleTime=dt
  Ruido de medida2 : RandomNumber  Variance=1e-6  Seed=123456  SampleTime=dt
  ym : Outport
  wires:
  y/1 -> Demux/1
  Ruido de medida1/1 -> Add2/1
  Add2/1 -> Mux2/1
  Demux/1 -> Add2/2
  Mux2/1 -> ym/1
  Demux/2 -> Add3/1
  Add3/1 -> Mux2/2
  Ruido de medida2/1 -> Add3/2

== system Simulink_6/Ejercicio 6/EJERCICIO 6 DISCRETO/Comparativa ejercicio 6/Comparativa modal/CONTROL LONGITUDINAL CONTINUA/ACTUADORES ==
  e : Inport
  Actuadores : Scope
  Demux : Demux  Outputs=2
  ELEVADOR : Subsystem
  Gain4 : Gain  Gain=[1 180/pi]
  Mux1 : Mux  Inputs=2
  THROTTLE : Subsystem
  u : Outport
  wires:
  Demux/1 -> THROTTLE/1(u_th)
  Demux/2 -> ELEVADOR/1(u_e)
  ELEVADOR/1(delta_e) -> Mux1/2
  e/1 -> Demux/1
  Mux1/1 -> u/1, Gain4/1
  Gain4/1 -> Actuadores/1
  THROTTLE/1(delta_th) -> Mux1/1

== system Simulink_6/Ejercicio 6/EJERCICIO 6 DISCRETO/Comparativa ejercicio 6/Comparativa modal/CONTROL LONGITUDINAL CONTINUA/DINAMICA LONGITUDINAL ==
  u : Inport
  Integrator5 : Integrator
  Km1 : Gain  Gain=D  Multiplication=Matrix(K*u)
  Km10 : Gain  Gain=A  Multiplication=Matrix(K*u)
  Km2 : Gain  Gain=C  Multiplication=Matrix(K*u)
  Km8 : Gain  Gain=B  Multiplication=Matrix(K*u)
  Sum1 : Sum  Inputs=++|
  Sum12 : Sum  Inputs=|++
  y : Outport
  wires:
  Km8/1 -> Sum12/1
  Sum12/1 -> Integrator5/1
  Integrator5/1 -> Km2/1, Km10/1  "x"
  Km10/1 -> Sum12/2
  Km2/1 -> Sum1/2
  Km1/1 -> Sum1/1
  Sum1/1 -> y/1
  u/1 -> Km8/1, Km1/1

== system Simulink_6/Ejercicio 6/EJERCICIO 6 DISCRETO/Comparativa ejercicio 6/Comparativa modal/CONTROL LONGITUDINAL CONTINUA/FILTRO SP ==
  vt-sp : Inport
  theta_sp : Inport  Port=2
  Mux4 : Mux  Inputs=2
  Rate Limiter : RateLimiter  RisingSlewLimit=3  FallingSlewLimit=-3  SampleTimeMode=inherited
  Transfer Fcn : TransferFcn  Denominator=[1 1]
  sp : Outport
  wires:
  Rate Limiter/1 -> Transfer Fcn/1
  Transfer Fcn/1 -> Mux4/1
  vt-sp/1 -> Rate Limiter/1
  Mux4/1 -> sp/1
  theta_sp/1 -> Mux4/2

== system Simulink_6/Ejercicio 6/EJERCICIO 6 DISCRETO/Comparativa ejercicio 6/Comparativa modal/CONTROL LONGITUDINAL CONTINUA/OBSERVADOR ==
  u : Inport
  y : Inport  Port=2
  Integrator5 : Integrator
  Km1 : Gain  Gain=D  Multiplication=Matrix(K*u)
  Km10 : Gain  Gain=A  Multiplication=Matrix(K*u)
  Km2 : Gain  Gain=C  Multiplication=Matrix(K*u)
  Km3 : Gain  Gain=Ko  Multiplication=Matrix(K*u)
  Km8 : Gain  Gain=B  Multiplication=Matrix(K*u)
  Sum1 : Sum  Inputs=++|
  Sum12 : Sum  Inputs=+++
  Sum2 : Sum  Inputs=+-|
  xest : Outport
  wires:
  Km8/1 -> Sum12/1
  Sum12/1 -> Integrator5/1
  Integrator5/1 -> Km2/1, Km10/1, xest/1  "xe"
  Km10/1 -> Sum12/3
  Km2/1 -> Sum1/2
  Km1/1 -> Sum1/1
  Sum1/1 -> Sum2/2  "ye"
  u/1 -> Km8/1, Km1/1
  y/1 -> Sum2/1
  Sum2/1 -> Km3/1
  Km3/1 -> Sum12/2

== system Simulink_6/Ejercicio 6/EJERCICIO 6 DISCRETO/Comparativa ejercicio 6/Comparativa modal/CONTROL LONGITUDINAL CONTINUA/SENSORES ==
  y : Inport
  Add2 : Sum
  Add3 : Sum
  Demux : Demux  Outputs=2
  Mux2 : Mux  Inputs=2
  Ruido de medida1 : RandomNumber  Variance=1e-6  Seed=123456  SampleTime=dt
  Ruido de medida2 : RandomNumber  Variance=1e-6  Seed=123456  SampleTime=dt
  ym : Outport
  wires:
  y/1 -> Demux/1
  Ruido de medida1/1 -> Add2/1
  Add2/1 -> Mux2/1
  Demux/1 -> Add2/2
  Mux2/1 -> ym/1
  Demux/2 -> Add3/1
  Add3/1 -> Mux2/2
  Ruido de medida2/1 -> Add3/2

== system Simulink_6/Ejercicio 6/EJERCICIO 6 DISCRETO/Comparativa ejercicio 6/Comparativa modal/CONTROL LONGITUDINAL DISCRETO/ACTUADORES ==
  e : Inport
  Actuadores : Scope
  Demux : Demux  Outputs=2
  ELEVADOR : Subsystem
  Gain4 : Gain  Gain=[1 180/pi]
  Mux1 : Mux  Inputs=2
  THROTTLE : Subsystem
  u : Outport
  wires:
  Demux/1 -> THROTTLE/1(u_th)
  Demux/2 -> ELEVADOR/1(u_e)
  ELEVADOR/1(delta_e) -> Mux1/2
  e/1 -> Demux/1
  Mux1/1 -> u/1, Gain4/1
  Gain4/1 -> Actuadores/1
  THROTTLE/1(delta_th) -> Mux1/1

== system Simulink_6/Ejercicio 6/EJERCICIO 6 DISCRETO/Comparativa ejercicio 6/Comparativa modal/CONTROL LONGITUDINAL DISCRETO/DINAMICA LONGITUDINAL ==
  u : Inport
  Integrator5 : Integrator
  Km1 : Gain  Gain=D  Multiplication=Matrix(K*u)
  Km10 : Gain  Gain=A  Multiplication=Matrix(K*u)
  Km2 : Gain  Gain=C  Multiplication=Matrix(K*u)
  Km8 : Gain  Gain=B  Multiplication=Matrix(K*u)
  Sum1 : Sum  Inputs=++|
  Sum12 : Sum  Inputs=|++
  y : Outport
  wires:
  Km8/1 -> Sum12/1
  Sum12/1 -> Integrator5/1
  Integrator5/1 -> Km2/1, Km10/1  "x"
  Km10/1 -> Sum12/2
  Km2/1 -> Sum1/2
  Km1/1 -> Sum1/1
  Sum1/1 -> y/1
  u/1 -> Km8/1, Km1/1

== system Simulink_6/Ejercicio 6/EJERCICIO 6 DISCRETO/Comparativa ejercicio 6/Comparativa modal/CONTROL LONGITUDINAL DISCRETO/FILTRO SP ==
  vt-sp : Inport
  theta_sp : Inport  Port=2
  Discrete Transfer Fcn : DiscreteTransferFcn  Numerator=[Tm]  Denominator=[1 -1+Tm]
  Mux4 : Mux  Inputs=2
  Rate Limiter : RateLimiter  RisingSlewLimit=3  FallingSlewLimit=-3  SampleTimeMode=inherited
  sp : Outport
  wires:
  Rate Limiter/1 -> Discrete Transfer Fcn/1
  vt-sp/1 -> Rate Limiter/1
  Mux4/1 -> sp/1
  theta_sp/1 -> Mux4/2
  Discrete Transfer Fcn/1 -> Mux4/1

== system Simulink_6/Ejercicio 6/EJERCICIO 6 DISCRETO/Comparativa ejercicio 6/Comparativa modal/CONTROL LONGITUDINAL DISCRETO/OBSERVADOR DISCRETO1 ==
  u(k) : Inport
  y(k) : Inport  Port=2
  Km1 : Gain  Gain=D  Multiplication=Matrix(K*u)
  Km10 : Gain  Gain=F  Multiplication=Matrix(K*u)
  Km2 : Gain  Gain=C  Multiplication=Matrix(K*u)
  Km3 : Gain  Gain=Ko  Multiplication=Matrix(K*u)
  Km8 : Gain  Gain=G  Multiplication=Matrix(K*u)
  Sum1 : Sum  Inputs=++|
  Sum12 : Sum  Inputs=+++
  Sum2 : Sum  Inputs=+-|
  Unit Delay : UnitDelay  SampleTime=Tm  HasFrameUpgradeWarning=on
  xe(k) : Outport
  wires:
  Km8/1 -> Sum12/1
  Sum12/1 -> Unit Delay/1  "xe(k+1)"
  Unit Delay/1 -> Km2/1, Km10/1, xe(k)/1  "xe(k)"
  Km10/1 -> Sum12/3
  Km2/1 -> Sum1/2
  Km1/1 -> Sum1/1
  Sum1/1 -> Sum2/2  "ye(k)"
  u(k)/1 -> Km8/1, Km1/1
  y(k)/1 -> Sum2/1
  Sum2/1 -> Km3/1
  Km3/1 -> Sum12/2

== system Simulink_6/Ejercicio 6/EJERCICIO 6 DISCRETO/Comparativa ejercicio 6/Comparativa modal/CONTROL LONGITUDINAL DISCRETO/sensor ==
  y : Inport
  Add2 : Sum
  Add3 : Sum
  Demux : Demux  Outputs=2
  Mux2 : Mux  Inputs=2
  Ruido de medida1 : RandomNumber  Variance=1e-6  Seed=123456  SampleTime=dt
  Ruido de medida2 : RandomNumber  Variance=1e-6  Seed=123456  SampleTime=dt
  ym : Outport
  wires:
  y/1 -> Demux/1
  Ruido de medida1/1 -> Add2/1
  Add2/1 -> Mux2/1
  Demux/1 -> Add2/2
  Mux2/1 -> ym/1
  Demux/2 -> Add3/1
  Add3/1 -> Mux2/2
  Ruido de medida2/1 -> Add3/2

== system Simulink_6/Ejercicio 6/EJERCICIO 6 DISCRETO/Comparativa ejercicio 7/Comparativa Integral/CONTROL LONGITUDINAL DISCRETO ACCION INTEGRAL/ACTUADORES ==
  e : Inport
  Actuadores : Scope
  Demux : Demux  Outputs=2
  ELEVADOR : Subsystem
  Gain4 : Gain  Gain=[1 180/pi]
  Mux1 : Mux  Inputs=2
  THROTTLE : Subsystem
  u : Outport
  wires:
  Demux/1 -> THROTTLE/1(u_th)
  Demux/2 -> ELEVADOR/1(u_e)
  ELEVADOR/1(delta_e) -> Mux1/2
  e/1 -> Demux/1
  Mux1/1 -> u/1, Gain4/1
  Gain4/1 -> Actuadores/1
  THROTTLE/1(delta_th) -> Mux1/1

== system Simulink_6/Ejercicio 6/EJERCICIO 6 DISCRETO/Comparativa ejercicio 7/Comparativa Integral/CONTROL LONGITUDINAL DISCRETO ACCION INTEGRAL/DINAMICA LONGITUDINAL ==
  u : Inport
  Integrator5 : Integrator
  Km1 : Gain  Gain=D  Multiplication=Matrix(K*u)
  Km10 : Gain  Gain=A  Multiplication=Matrix(K*u)
  Km2 : Gain  Gain=C  Multiplication=Matrix(K*u)
  Km8 : Gain  Gain=B  Multiplication=Matrix(K*u)
  Sum1 : Sum  Inputs=++|
  Sum12 : Sum  Inputs=|++
  y : Outport
  wires:
  Km8/1 -> Sum12/1
  Sum12/1 -> Integrator5/1
  Integrator5/1 -> Km2/1, Km10/1  "x"
  Km10/1 -> Sum12/2
  Km2/1 -> Sum1/2
  Km1/1 -> Sum1/1
  Sum1/1 -> y/1
  u/1 -> Km8/1, Km1/1

== system Simulink_6/Ejercicio 6/EJERCICIO 6 DISCRETO/Comparativa ejercicio 7/Comparativa Integral/CONTROL LONGITUDINAL DISCRETO ACCION INTEGRAL/FILTRO SP ==
  vt-sp : Inport
  theta_sp : Inport  Port=2
  Discrete Transfer Fcn : DiscreteTransferFcn  Numerator=[Tm]  Denominator=[1 -1+Tm]
  Mux4 : Mux  Inputs=2
  Rate Limiter : RateLimiter  RisingSlewLimit=3  FallingSlewLimit=-3  SampleTimeMode=inherited
  sp : Outport
  wires:
  vt-sp/1 -> Rate Limiter/1
  Mux4/1 -> sp/1
  theta_sp/1 -> Mux4/2
  Rate Limiter/1 -> Discrete Transfer Fcn/1
  Discrete Transfer Fcn/1 -> Mux4/1

== system Simulink_6/Ejercicio 6/EJERCICIO 6 DISCRETO/Comparativa ejercicio 7/Comparativa Integral/CONTROL LONGITUDINAL DISCRETO ACCION INTEGRAL/OBSERVADOR DISCRETO ==
  u(k) : Inport
  y(k) : Inport  Port=2
  Km1 : Gain  Gain=D  Multiplication=Matrix(K*u)
  Km10 : Gain  Gain=F  Multiplication=Matrix(K*u)
  Km2 : Gain  Gain=C  Multiplication=Matrix(K*u)
  Km3 : Gain  Gain=Ko  Multiplication=Matrix(K*u)
  Km8 : Gain  Gain=G  Multiplication=Matrix(K*u)
  Sum1 : Sum  Inputs=++|
  Sum12 : Sum  Inputs=+++
  Sum2 : Sum  Inputs=+-|
  Unit Delay : UnitDelay  SampleTime=Tm  HasFrameUpgradeWarning=on
  xe(k) : Outport
  wires:
  Km8/1 -> Sum12/1
  Sum12/1 -> Unit Delay/1  "xe(k+1)"
  Unit Delay/1 -> Km2/1, Km10/1, xe(k)/1  "xe(k)"
  Km10/1 -> Sum12/3
  Km2/1 -> Sum1/2
  Km1/1 -> Sum1/1
  Sum1/1 -> Sum2/2  "ye(k)"
  u(k)/1 -> Km8/1, Km1/1
  y(k)/1 -> Sum2/1
  Sum2/1 -> Km3/1
  Km3/1 -> Sum12/2

== system Simulink_6/Ejercicio 6/EJERCICIO 6 DISCRETO/Comparativa ejercicio 7/Comparativa Integral/CONTROL LONGITUDINAL DISCRETO ACCION INTEGRAL/SENSORES ==
  y : Inport
  Add2 : Sum
  Add3 : Sum
  Demux : Demux  Outputs=2
  Mux2 : Mux  Inputs=2
  Ruido de medida1 : RandomNumber  Variance=1e-6  Seed=123456  SampleTime=dt
  Ruido de medida2 : RandomNumber  Variance=1e-6  Seed=123456  SampleTime=dt
  ym : Outport
  wires:
  y/1 -> Demux/1
  Ruido de medida1/1 -> Add2/1
  Add2/1 -> Mux2/1
  Demux/1 -> Add2/2
  Mux2/1 -> ym/1
  Demux/2 -> Add3/1
  Add3/1 -> Mux2/2
  Ruido de medida2/1 -> Add3/2

== system Simulink_6/Ejercicio 6/EJERCICIO 6 DISCRETO/Comparativa ejercicio 7/Comparativa Integral/CONTROL LONGITUDINAL DISCRETO ACCION INTEGRAL1/ACTUADORES ==
  e : Inport
  Actuadores : Scope
  Demux : Demux  Outputs=2
  ELEVADOR : Subsystem
  Gain4 : Gain  Gain=[1 180/pi]
  Mux1 : Mux  Inputs=2
  THROTTLE : Subsystem
  u : Outport
  wires:
  Demux/1 -> THROTTLE/1(u_th)
  Demux/2 -> ELEVADOR/1(u_e)
  ELEVADOR/1(delta_e) -> Mux1/2
  e/1 -> Demux/1
  Mux1/1 -> u/1, Gain4/1
  Gain4/1 -> Actuadores/1
  THROTTLE/1(delta_th) -> Mux1/1

== system Simulink_6/Ejercicio 6/EJERCICIO 6 DISCRETO/Comparativa ejercicio 7/Comparativa Integral/CONTROL LONGITUDINAL DISCRETO ACCION INTEGRAL1/DINAMICA LONGITUDINAL ==
  u : Inport
  Integrator5 : Integrator
  Km1 : Gain  Gain=D  Multiplication=Matrix(K*u)
  Km10 : Gain  Gain=A  Multiplication=Matrix(K*u)
  Km2 : Gain  Gain=C  Multiplication=Matrix(K*u)
  Km8 : Gain  Gain=B  Multiplication=Matrix(K*u)
  Sum1 : Sum  Inputs=++|
  Sum12 : Sum  Inputs=|++
  y : Outport
  wires:
  Km8/1 -> Sum12/1
  Sum12/1 -> Integrator5/1
  Integrator5/1 -> Km2/1, Km10/1  "x"
  Km10/1 -> Sum12/2
  Km2/1 -> Sum1/2
  Km1/1 -> Sum1/1
  Sum1/1 -> y/1
  u/1 -> Km8/1, Km1/1

== system Simulink_6/Ejercicio 6/EJERCICIO 6 DISCRETO/Comparativa ejercicio 7/Comparativa Integral/CONTROL LONGITUDINAL DISCRETO ACCION INTEGRAL1/FILTRO SP ==
  vt-sp : Inport
  theta_sp : Inport  Port=2
  Discrete Transfer Fcn : DiscreteTransferFcn  Numerator=[Tm]  Denominator=[1 -1+Tm]
  Mux4 : Mux  Inputs=2
  Rate Limiter : RateLimiter  RisingSlewLimit=3  FallingSlewLimit=-3  SampleTimeMode=inherited
  sp : Outport
  wires:
  vt-sp/1 -> Rate Limiter/1
  Mux4/1 -> sp/1
  theta_sp/1 -> Mux4/2
  Rate Limiter/1 -> Discrete Transfer Fcn/1
  Discrete Transfer Fcn/1 -> Mux4/1

== system Simulink_6/Ejercicio 6/EJERCICIO 6 DISCRETO/Comparativa ejercicio 7/Comparativa Integral/CONTROL LONGITUDINAL DISCRETO ACCION INTEGRAL1/OBSERVADOR DISCRETO ==
  u(k) : Inport
  y(k) : Inport  Port=2
  Km1 : Gain  Gain=D  Multiplication=Matrix(K*u)
  Km10 : Gain  Gain=F  Multiplication=Matrix(K*u)
  Km2 : Gain  Gain=C  Multiplication=Matrix(K*u)
  Km3 : Gain  Gain=Ko  Multiplication=Matrix(K*u)
  Km8 : Gain  Gain=G  Multiplication=Matrix(K*u)
  Sum1 : Sum  Inputs=++|
  Sum12 : Sum  Inputs=+++
  Sum2 : Sum  Inputs=+-|
  Unit Delay : UnitDelay  SampleTime=Tm  HasFrameUpgradeWarning=on
  xe(k) : Outport
  wires:
  Km8/1 -> Sum12/1
  Sum12/1 -> Unit Delay/1  "xe(k+1)"
  Unit Delay/1 -> Km2/1, Km10/1, xe(k)/1  "xe(k)"
  Km10/1 -> Sum12/3
  Km2/1 -> Sum1/2
  Km1/1 -> Sum1/1
  Sum1/1 -> Sum2/2  "ye(k)"
  u(k)/1 -> Km8/1, Km1/1
  y(k)/1 -> Sum2/1
  Sum2/1 -> Km3/1
  Km3/1 -> Sum12/2

== system Simulink_6/Ejercicio 6/EJERCICIO 6 DISCRETO/Comparativa ejercicio 7/Comparativa Integral/CONTROL LONGITUDINAL DISCRETO ACCION INTEGRAL1/SENSORES ==
  y : Inport
  Add2 : Sum
  Add3 : Sum
  Demux : Demux  Outputs=2
  Mux2 : Mux  Inputs=2
  Ruido de medida1 : RandomNumber  Variance=1e-6  Seed=123456  SampleTime=dt
  Ruido de medida2 : RandomNumber  Variance=1e-6  Seed=123456  SampleTime=dt
  ym : Outport
  wires:
  y/1 -> Demux/1
  Ruido de medida1/1 -> Add2/1
  Add2/1 -> Mux2/1
  Demux/1 -> Add2/2
  Mux2/1 -> ym/1
  Demux/2 -> Add3/1
  Add3/1 -> Mux2/2
  Ruido de medida2/1 -> Add3/2

== system Simulink_6/Ejercicio 6/EJERCICIO 6 DISCRETO/Comparativa ejercicio 7/Comparativa modal/CONTROL LONGITUDINAL DISCRETO EJERCICIO 6/ACTUADORES ==
  e : Inport
  Actuadores : Scope
  Demux : Demux  Outputs=2
  ELEVADOR : Subsystem
  Gain4 : Gain  Gain=[1 180/pi]
  Mux1 : Mux  Inputs=2
  THROTTLE : Subsystem
  u : Outport
  wires:
  Demux/1 -> THROTTLE/1(u_th)
  Demux/2 -> ELEVADOR/1(u_e)
  ELEVADOR/1(delta_e) -> Mux1/2
  e/1 -> Demux/1
  Mux1/1 -> u/1, Gain4/1
  Gain4/1 -> Actuadores/1
  THROTTLE/1(delta_th) -> Mux1/1

== system Simulink_6/Ejercicio 6/EJERCICIO 6 DISCRETO/Comparativa ejercicio 7/Comparativa modal/CONTROL LONGITUDINAL DISCRETO EJERCICIO 6/DINAMICA LONGITUDINAL ==
  u : Inport
  Integrator5 : Integrator
  Km1 : Gain  Gain=D  Multiplication=Matrix(K*u)
  Km10 : Gain  Gain=A  Multiplication=Matrix(K*u)
  Km2 : Gain  Gain=C  Multiplication=Matrix(K*u)
  Km8 : Gain  Gain=B  Multiplication=Matrix(K*u)
  Sum1 : Sum  Inputs=++|
  Sum12 : Sum  Inputs=|++
  y : Outport
  wires:
  Km8/1 -> Sum12/1
  Sum12/1 -> Integrator5/1
  Integrator5/1 -> Km2/1, Km10/1  "x"
  Km10/1 -> Sum12/2
  Km2/1 -> Sum1/2
  Km1/1 -> Sum1/1
  Sum1/1 -> y/1
  u/1 -> Km8/1, Km1/1

== system Simulink_6/Ejercicio 6/EJERCICIO 6 DISCRETO/Comparativa ejercicio 7/Comparativa modal/CONTROL LONGITUDINAL DISCRETO EJERCICIO 6/FILTRO SP ==
  vt-sp : Inport
  theta_sp : Inport  Port=2
  Discrete Transfer Fcn : DiscreteTransferFcn  Numerator=[Tm]  Denominator=[1 -1+Tm]
  Mux4 : Mux  Inputs=2
  Rate Limiter : RateLimiter  RisingSlewLimit=3  FallingSlewLimit=-3  SampleTimeMode=inherited
  sp : Outport
  wires:
  Rate Limiter/1 -> Discrete Transfer Fcn/1
  vt-sp/1 -> Rate Limiter/1
  Mux4/1 -> sp/1
  theta_sp/1 -> Mux4/2
  Discrete Transfer Fcn/1 -> Mux4/1

== system Simulink_6/Ejercicio 6/EJERCICIO 6 DISCRETO/Comparativa ejercicio 7/Comparativa modal/CONTROL LONGITUDINAL DISCRETO EJERCICIO 6/OBSERVADOR DISCRETO1 ==
  u(k) : Inport
  y(k) : Inport  Port=2
  Km1 : Gain  Gain=D  Multiplication=Matrix(K*u)
  Km10 : Gain  Gain=F  Multiplication=Matrix(K*u)
  Km2 : Gain  Gain=C  Multiplication=Matrix(K*u)
  Km3 : Gain  Gain=Ko  Multiplication=Matrix(K*u)
  Km8 : Gain  Gain=G  Multiplication=Matrix(K*u)
  Sum1 : Sum  Inputs=++|
  Sum12 : Sum  Inputs=+++
  Sum2 : Sum  Inputs=+-|
  Unit Delay : UnitDelay  SampleTime=Tm  HasFrameUpgradeWarning=on
  xe(k) : Outport
  wires:
  Km8/1 -> Sum12/1
  Sum12/1 -> Unit Delay/1  "xe(k+1)"
  Unit Delay/1 -> Km2/1, Km10/1, xe(k)/1  "xe(k)"
  Km10/1 -> Sum12/3
  Km2/1 -> Sum1/2
  Km1/1 -> Sum1/1
  Sum1/1 -> Sum2/2  "ye(k)"
  u(k)/1 -> Km8/1, Km1/1
  y(k)/1 -> Sum2/1
  Sum2/1 -> Km3/1
  Km3/1 -> Sum12/2

== system Simulink_6/Ejercicio 6/EJERCICIO 6 DISCRETO/Comparativa ejercicio 7/Comparativa modal/CONTROL LONGITUDINAL DISCRETO EJERCICIO 6/sensor ==
  y : Inport
  Add2 : Sum
  Add3 : Sum
  Demux : Demux  Outputs=2
  Mux2 : Mux  Inputs=2
  Ruido de medida1 : RandomNumber  Variance=1e-6  Seed=123456  SampleTime=dt
  Ruido de medida2 : RandomNumber  Variance=1e-6  Seed=123456  SampleTime=dt
  ym : Outport
  wires:
  y/1 -> Demux/1
  Ruido de medida1/1 -> Add2/1
  Add2/1 -> Mux2/1
  Demux/1 -> Add2/2
  Mux2/1 -> ym/1
  Demux/2 -> Add3/1
  Add3/1 -> Mux2/2
  Ruido de medida2/1 -> Add3/2

== system Simulink_6/Ejercicio 6/EJERCICIO 6 DISCRETO/Comparativa ejercicio 7/Comparativa modal/CONTROL LONGITUDINAL DISCRETO EJERCICIO 7/ACTUADORES ==
  e : Inport
  Actuadores : Scope
  Demux : Demux  Outputs=2
  ELEVADOR : Subsystem
  Gain4 : Gain  Gain=[1 180/pi]
  Mux1 : Mux  Inputs=2
  THROTTLE : Subsystem
  u : Outport
  wires:
  Demux/1 -> THROTTLE/1(u_th)
  Demux/2 -> ELEVADOR/1(u_e)
  ELEVADOR/1(delta_e) -> Mux1/2
  e/1 -> Demux/1
  Mux1/1 -> u/1, Gain4/1
  Gain4/1 -> Actuadores/1
  THROTTLE/1(delta_th) -> Mux1/1

== system Simulink_6/Ejercicio 6/EJERCICIO 6 DISCRETO/Comparativa ejercicio 7/Comparativa modal/CONTROL LONGITUDINAL DISCRETO EJERCICIO 7/DINAMICA LONGITUDINAL ==
  u : Inport
  Integrator5 : Integrator
  Km1 : Gain  Gain=D  Multiplication=Matrix(K*u)
  Km10 : Gain  Gain=A  Multiplication=Matrix(K*u)
  Km2 : Gain  Gain=C  Multiplication=Matrix(K*u)
  Km8 : Gain  Gain=B  Multiplication=Matrix(K*u)
  Sum1 : Sum  Inputs=++|
  Sum12 : Sum  Inputs=|++
  y : Outport
  wires:
  Km8/1 -> Sum12/1
  Sum12/1 -> Integrator5/1
  Integrator5/1 -> Km2/1, Km10/1  "x"
  Km10/1 -> Sum12/2
  Km2/1 -> Sum1/2
  Km1/1 -> Sum1/1
  Sum1/1 -> y/1
  u/1 -> Km8/1, Km1/1

== system Simulink_6/Ejercicio 6/EJERCICIO 6 DISCRETO/Comparativa ejercicio 7/Comparativa modal/CONTROL LONGITUDINAL DISCRETO EJERCICIO 7/FILTRO SP ==
  vt-sp : Inport
  theta_sp : Inport  Port=2
  Discrete Transfer Fcn : DiscreteTransferFcn  Numerator=[Tm]  Denominator=[1 -1+Tm]
  Mux4 : Mux  Inputs=2
  Rate Limiter : RateLimiter  RisingSlewLimit=3  FallingSlewLimit=-3  SampleTimeMode=inherited
  sp : Outport
  wires:
  Rate Limiter/1 -> Discrete Transfer Fcn/1
  vt-sp/1 -> Rate Limiter/1
  Mux4/1 -> sp/1
  theta_sp/1 -> Mux4/2
  Discrete Transfer Fcn/1 -> Mux4/1

== system Simulink_6/Ejercicio 6/EJERCICIO 6 DISCRETO/Comparativa ejercicio 7/Comparativa modal/CONTROL LONGITUDINAL DISCRETO EJERCICIO 7/OBSERVADOR DISCRETO1 ==
  u(k) : Inport
  y(k) : Inport  Port=2
  Km1 : Gain  Gain=D  Multiplication=Matrix(K*u)
  Km10 : Gain  Gain=F  Multiplication=Matrix(K*u)
  Km2 : Gain  Gain=C  Multiplication=Matrix(K*u)
  Km3 : Gain  Gain=Ko  Multiplication=Matrix(K*u)
  Km8 : Gain  Gain=G  Multiplication=Matrix(K*u)
  Sum1 : Sum  Inputs=++|
  Sum12 : Sum  Inputs=+++
  Sum2 : Sum  Inputs=+-|
  Unit Delay : UnitDelay  SampleTime=Tm  HasFrameUpgradeWarning=on
  xe(k) : Outport
  wires:
  Km8/1 -> Sum12/1
  Sum12/1 -> Unit Delay/1  "xe(k+1)"
  Unit Delay/1 -> Km2/1, Km10/1, xe(k)/1  "xe(k)"
  Km10/1 -> Sum12/3
  Km2/1 -> Sum1/2
  Km1/1 -> Sum1/1
  Sum1/1 -> Sum2/2  "ye(k)"
  u(k)/1 -> Km8/1, Km1/1
  y(k)/1 -> Sum2/1
  Sum2/1 -> Km3/1
  Km3/1 -> Sum12/2

== system Simulink_6/Ejercicio 6/EJERCICIO 6 DISCRETO/Comparativa ejercicio 7/Comparativa modal/CONTROL LONGITUDINAL DISCRETO EJERCICIO 7/sensor ==
  y : Inport
  Add2 : Sum
  Add3 : Sum
  Demux : Demux  Outputs=2
  Mux2 : Mux  Inputs=2
  Ruido de medida1 : RandomNumber  Variance=1e-6  Seed=123456  SampleTime=dt
  Ruido de medida2 : RandomNumber  Variance=1e-6  Seed=123456  SampleTime=dt
  ym : Outport
  wires:
  y/1 -> Demux/1
  Ruido de medida1/1 -> Add2/1
  Add2/1 -> Mux2/1
  Demux/1 -> Add2/2
  Mux2/1 -> ym/1
  Demux/2 -> Add3/1
  Add3/1 -> Mux2/2
  Ruido de medida2/1 -> Add3/2

== system Simulink_6/Ejercicio 6/EJERCICIO 6 DISCRETO/Comparativa ejercicio 6/Comparativa Integral/CONTROL LONGITUDINAL CONTINUO ACCION INTEGRAL/ACTUADORES/ELEVADOR ==
  u_e : Inport
  Fpdot1 : Saturate  UpperLimit=delta_e_dot_lim(2)  LowerLimit=delta_e_dot_lim(1)
  Integrator4 : Integrator  LimitOutput=on  UpperSaturationLimit=delta_e_lim(2)  LowerSaturationLimit=delta_e_lim(1)
  KT/taup3 : Gain  Gain=1/tau_e
  Km9 : Gain  Gain=1/tau_e
  Sum10 : Sum  Inputs=|+-
  delta_e : Outport
  wires:
  Km9/1 -> Sum10/2
  Integrator4/1 -> Km9/1, delta_e/1  "delta_e"
  Sum10/1 -> Fpdot1/1  "delta_e_dot"
  KT/taup3/1 -> Sum10/1
  Fpdot1/1 -> Integrator4/1
  u_e/1 -> KT/taup3/1

== system Simulink_6/Ejercicio 6/EJERCICIO 6 DISCRETO/Comparativa ejercicio 6/Comparativa Integral/CONTROL LONGITUDINAL CONTINUO ACCION INTEGRAL/ACTUADORES/THROTTLE ==
  u_th : Inport
  Fpdot1 : Saturate  UpperLimit=delta_th_dot_lim(2)  LowerLimit=delta_th_dot_lim(1)
  Integrator4 : Integrator  LimitOutput=on  UpperSaturationLimit=delta_th_lim(2)  LowerSaturationLimit=delta_th_lim(1)
  KT/taup3 : Gain  Gain=1/tau_th
  Km9 : Gain  Gain=1/tau_th
  Sum10 : Sum  Inputs=|+-
  delta_th : Outport
  wires:
  Km9/1 -> Sum10/2
  Integrator4/1 -> Km9/1, delta_th/1  "delta_th"
  Sum10/1 -> Fpdot1/1  "delta_th_dot"
  KT/taup3/1 -> Sum10/1
  Fpdot1/1 -> Integrator4/1
  u_th/1 -> KT/taup3/1

== system Simulink_6/Ejercicio 6/EJERCICIO 6 DISCRETO/Comparativa ejercicio 6/Comparativa Integral/CONTROL LONGITUDINAL DISCRETO ACCION INTEGRAL/ACTUADORES/ELEVADOR ==
  u_e : Inport
  Fpdot1 : Saturate  UpperLimit=delta_e_dot_lim(2)  LowerLimit=delta_e_dot_lim(1)
  Integrator4 : Integrator  LimitOutput=on  UpperSaturationLimit=delta_e_lim(2)  LowerSaturationLimit=delta_e_lim(1)
  KT/taup3 : Gain  Gain=1/tau_e
  Km9 : Gain  Gain=1/tau_e
  Sum10 : Sum  Inputs=|+-
  delta_e : Outport
  wires:
  Km9/1 -> Sum10/2
  Integrator4/1 -> Km9/1, delta_e/1  "delta_e"
  Sum10/1 -> Fpdot1/1  "delta_e_dot"
  KT/taup3/1 -> Sum10/1
  Fpdot1/1 -> Integrator4/1
  u_e/1 -> KT/taup3/1

== system Simulink_6/Ejercicio 6/EJERCICIO 6 DISCRETO/Comparativa ejercicio 6/Comparativa Integral/CONTROL LONGITUDINAL DISCRETO ACCION INTEGRAL/ACTUADORES/THROTTLE ==
  u_th : Inport
  Fpdot1 : Saturate  UpperLimit=delta_th_dot_lim(2)  LowerLimit=delta_th_dot_lim(1)
  Integrator4 : Integrator  LimitOutput=on  UpperSaturationLimit=delta_th_lim(2)  LowerSaturationLimit=delta_th_lim(1)
  KT/taup3 : Gain  Gain=1/tau_th
  Km9 : Gain  Gain=1/tau_th
  Sum10 : Sum  Inputs=|+-
  delta_th : Outport
  wires:
  Km9/1 -> Sum10/2
  Integrator4/1 -> Km9/1, delta_th/1  "delta_th"
  Sum10/1 -> Fpdot1/1  "delta_th_dot"
  KT/taup3/1 -> Sum10/1
  Fpdot1/1 -> Integrator4/1
  u_th/1 -> KT/taup3/1
